simulink model "Quad_tilt_dynamic_fl"  (R2017b)
settings: Solver=FixedStepAuto  StartTime=0.0  StopTime=30  FixedStep=0.0001  RelTol=1e-3
values from neighbouring files (symbols this model uses):
  alpha1_0 = 0.0    (= 0)    [parameters_quad_tilt_dynamic.m]
  alpha2_0 = pi    (= 3.14159265359)    [parameters_quad_tilt_dynamic.m]
  alpha3_0 = 0.0    (= 0)    [parameters_quad_tilt_dynamic.m]
  alpha4_0 = pi    (= 3.14159265359)    [parameters_quad_tilt_dynamic.m]
  d2wd = zeros(3,1)    [parameters_quad_tilt_dynamic.m]
  dx0 = 0.0    (= 0)    [parameters_quad_tilt_dynamic.m]
  dy0 = 0.0    (= 0)    [parameters_quad_tilt_dynamic.m]
  dz0 = 1.0    (= 1)    [parameters_quad_tilt_dynamic.m]
  gravity = [0.0;0.0;-g]    [parameters_quad_tilt_dynamic.m]
  Inertia_Matrix = [Ix, 0,  0 ... (first row only)    [parameters_quad_tilt_dynamic.m]
  Inv_Iner = inv(Inertia_Matrix)    [parameters_quad_tilt_dynamic.m]
  K2d = eye(3) * 7.5    [parameters_quad_tilt_dynamic.m]
  Kd = eye(3) * 25.75    [parameters_quad_tilt_dynamic.m]
  kf = 0.3    [parameters_quad_tilt_dynamic.m]
  km = 0.1    [parameters_quad_tilt_dynamic.m]
  Kp = eye(3) * 15    [parameters_quad_tilt_dynamic.m]
  Kw = eye(3) * 10    [parameters_quad_tilt_dynamic.m]
  l = 0.1    [parameters_quad_tilt_dynamic.m]
  m = 0.650    (= 0.65)    [parameters_quad_tilt_dynamic.m]
  Rb0 = eye(3)    [parameters_quad_tilt_dynamic.m]
  Rd = [  1.0000000,  0.0000000,  0.0000000 ... (first row only)    [parameters_quad_tilt_dynamic.m]
  Wb0 = [0.0, 0.0, 0.0]    [parameters_quad_tilt_dynamic.m]
  x0 = 1.0    (= 1)    [parameters_quad_tilt_dynamic.m]
  y0 = 0.0    (= 0)    [parameters_quad_tilt_dynamic.m]
  z0 = 0.0    (= 0)    [parameters_quad_tilt_dynamic.m]
libraries: simulink x4
settings Model: Creator=Marco  LastModifiedBy=Marco
settings CodeAppCC: StateflowObjectComments=on

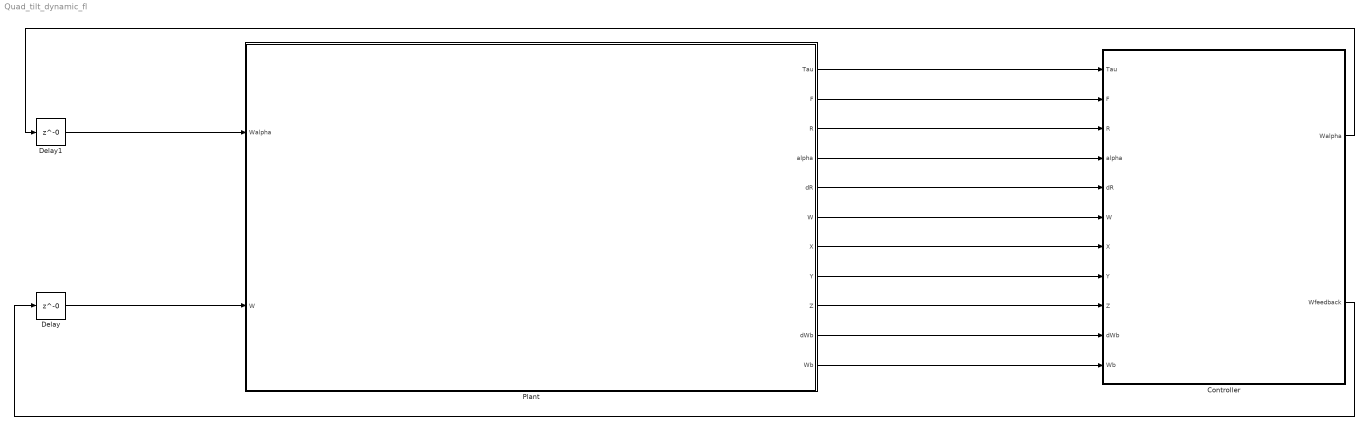
== system Quad_tilt_dynamic_fl ==
  Controller : Subsystem
  Delay : Delay  DelayLength=0  InitialCondition=zeros(4,1)
  Delay1 : Delay  DelayLength=0  InitialCondition=zeros(4,1)
  Plant : Subsystem
  wires:
  Delay/1 -> Plant/2(W)
  Delay1/1 -> Plant/1("Walpha ")
  Plant/1(Tau) -> Controller/1(Tau)
  Plant/2(F) -> Controller/2(F)
  Plant/3(R) -> Controller/3(R)
  Plant/4(alpha) -> Controller/4(alpha)
  Plant/6("W ") -> Controller/6(W)
  Plant/5(dR) -> Controller/5(dR)
  Plant/7(X) -> Controller/7(X)
  Plant/8(Y) -> Controller/8(Y)
  Plant/9(Z) -> Controller/9(Z)
  Controller/1(Walpha) -> Delay1/1
  Controller/2(Wfeedback) -> Delay/1
  Plant/10(dWb) -> Controller/10(dWb)
  Plant/11(Wb) -> Controller/11(Wb)

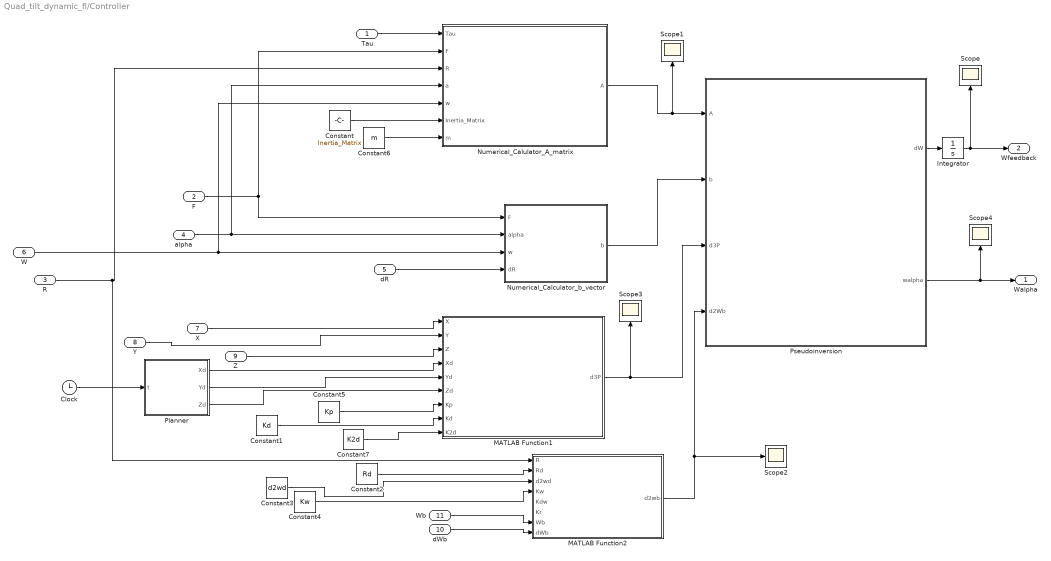
== system Quad_tilt_dynamic_fl/Controller ==
  Tau : Inport
  F : Inport  Port=2
  R : Inport  Port=3
  alpha : Inport  Port=4
  dR : Inport  Port=5
  W : Inport  Port=6
  X : Inport  Port=7
  Y : Inport  Port=8
  Z : Inport  Port=9
  dWb : Inport  Port=10
  Wb : Inport  Port=11
  Clock : Clock
  Constant : Constant  Value=Inertia_Matrix
  Constant1 : Constant  Value=Kd
  Constant2 : Constant  Value=Rd
  Constant3 : Constant  Value=d2wd
  Constant4 : Constant  Value=Kw
  Constant5 : Constant  Value=Kp
  Constant6 : Constant  Value=m
  Constant7 : Constant  Value=K2d
  Integrator : Integrator  InitialCondition=zeros(4,1)
  MATLAB Function1 : MATLAB Function  TreatAsAtomicUnit=on
  MATLAB Function2 : MATLAB Function  TreatAsAtomicUnit=on
  Numerical_Calculator_b_vector : MATLAB Function  TreatAsAtomicUnit=on
  Numerical_Calulator_A_matrix : MATLAB Function  TreatAsAtomicUnit=on
  Planner : MATLAB Function  TreatAsAtomicUnit=on
  Pseudoinversion : MATLAB Function  TreatAsAtomicUnit=on
  Scope{,1..4} (5 alike) : Scope
  Walpha : Outport
  Wfeedback : Outport  Port=2
  wires:
  Tau/1 -> Numerical_Calulator_A_matrix/1(Tau)
  alpha/1 -> Numerical_Calculator_b_vector/2(alpha), Numerical_Calulator_A_matrix/4(a)
  W/1 -> Numerical_Calculator_b_vector/3(w), Numerical_Calulator_A_matrix/5(w)
  R/1 -> MATLAB Function2/1(R), Numerical_Calulator_A_matrix/3(R)
  dR/1 -> Numerical_Calculator_b_vector/4(dR)
  F/1 -> Numerical_Calculator_b_vector/1(F), Numerical_Calulator_A_matrix/2(F)
  Constant/1 -> Numerical_Calulator_A_matrix/6(Inertia_Matrix)
  X/1 -> MATLAB Function1/1(X)
  Y/1 -> MATLAB Function1/2(Y)
  Z/1 -> MATLAB Function1/3(Z)
  Constant5/1 -> MATLAB Function1/7(Kp)
  Constant1/1 -> MATLAB Function1/8(Kd)
  Clock/1 -> Planner/1(t)
  Planner/1(Xd) -> MATLAB Function1/4(Xd)
  Planner/2(Yd) -> MATLAB Function1/5(Yd)
  Planner/3(Zd) -> MATLAB Function1/6(Zd)
  Constant3/1 -> MATLAB Function2/3(d2wd)
  Constant2/1 -> MATLAB Function2/2(Rd)
  Constant4/1 -> MATLAB Function2/4(Kw)
  Numerical_Calculator_b_vector/1(b) -> Pseudoinversion/2(b)
  Numerical_Calulator_A_matrix/1(A) -> Pseudoinversion/1(A), Scope1/1
  MATLAB Function1/1(d3P) -> Scope3/1, Pseudoinversion/3(d3P)
  Pseudoinversion/1(dW) -> Integrator/1
  Pseudoinversion/2(walpha) -> Scope4/1, Walpha/1
  Integrator/1 -> Scope/1, Wfeedback/1
  MATLAB Function2/1(d2wb) -> Scope2/1, Pseudoinversion/4(d2Wb)
  Constant6/1 -> Numerical_Calulator_A_matrix/7(m)
  Constant7/1 -> MATLAB Function1/9(K2d)
  Wb/1 -> MATLAB Function2/7(Wb)
  dWb/1 -> MATLAB Function2/8(dWb)

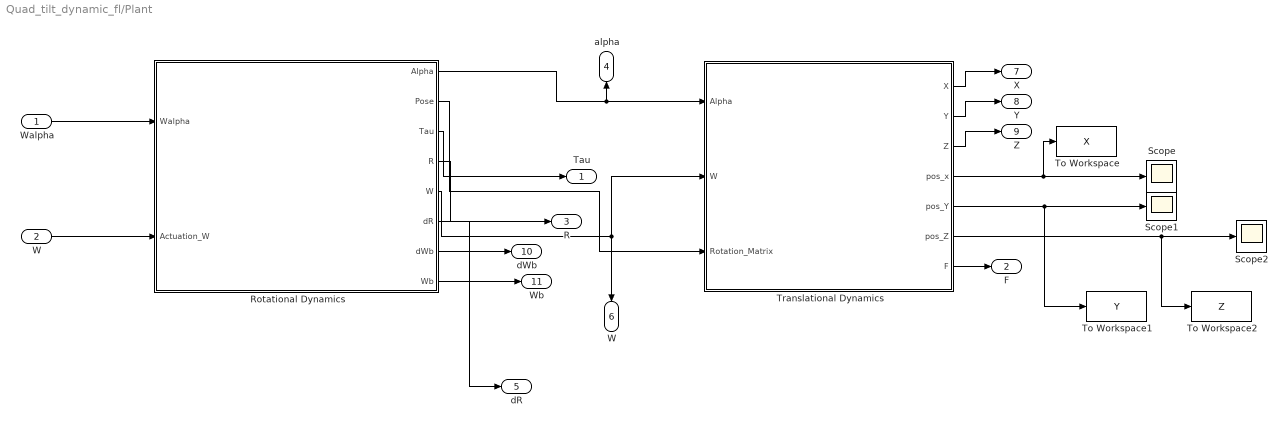
== system Quad_tilt_dynamic_fl/Plant ==
  "Walpha " : Inport
  W : Inport  Port=2
  Rotational Dynamics : Subsystem
  Scope : Scope
  Scope1 : Scope
  Scope2 : Scope
  To Workspace : ToWorkspace  VariableName=X  SampleTime=-1
  To Workspace1 : ToWorkspace  VariableName=Y  SampleTime=-1
  To Workspace2 : ToWorkspace  VariableName=Z  SampleTime=-1
  Translational Dynamics : Subsystem
  Tau : Outport
  F : Outport  Port=2
  R : Outport  Port=3
  alpha : Outport  Port=4
  dR : Outport  Port=5
  "W " : Outport  Port=6
  X : Outport  Port=7
  Y : Outport  Port=8
  Z : Outport  Port=9
  dWb : Outport  Port=10
  Wb : Outport  Port=11
  wires:
  Rotational Dynamics/3(Tau) -> Tau/1
  Rotational Dynamics/2(Pose) -> Translational Dynamics/3(Rotation_Matrix)
  Rotational Dynamics/1(Alpha) -> alpha/1, Translational Dynamics/1(Alpha)
  Translational Dynamics/7(F) -> F/1
  Translational Dynamics/1(X) -> X/1
  Translational Dynamics/2(Y) -> Y/1
  Translational Dynamics/3(Z) -> Z/1
  Rotational Dynamics/4(R) -> R/1
  "Walpha "/1 -> Rotational Dynamics/1(Walpha)
  W/1 -> Rotational Dynamics/2(Actuation_W)
  Rotational Dynamics/5(W) -> Translational Dynamics/2(W), "W "/1
  Translational Dynamics/4(pos_x) -> To Workspace/1, Scope/1
  Translational Dynamics/5(pos_Y) -> To Workspace1/1, Scope1/1
  Translational Dynamics/6(pos_Z) -> To Workspace2/1, Scope2/1
  Rotational Dynamics/6(dR) -> dR/1
  Rotational Dynamics/7(dWb) -> dWb/1
  Rotational Dynamics/8(Wb) -> Wb/1

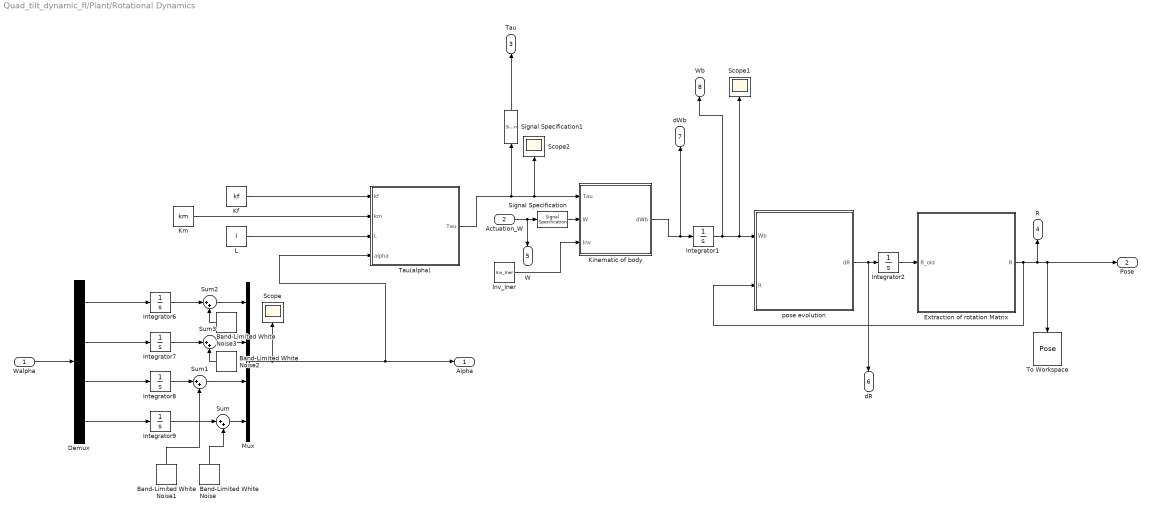
== system Quad_tilt_dynamic_fl/Plant/Rotational Dynamics ==
  Walpha : Inport
  Actuation_W : Inport  Port=2
  Band-Limited White Noise : simulink/Sources/Band-Limited White Noise  Cov=[0]  Ts=0.1  seed=[23345431]
  Band-Limited White Noise1 : simulink/Sources/Band-Limited White Noise  Cov=[0]  Ts=0.1  seed=[233423781]
  Band-Limited White Noise2 : simulink/Sources/Band-Limited White Noise  Cov=[0]  Ts=0.1  seed=[232441]
  Band-Limited White Noise3 : simulink/Sources/Band-Limited White Noise  Cov=[0]  Ts=0.1  seed=[23341]
  Demux : Demux
  Extraction of rotation Matrix : MATLAB Function  TreatAsAtomicUnit=on
  Integrator1 : Integrator  InitialCondition=Wb0
  Integrator2 : Integrator  InitialCondition=Rb0
  Integrator6 : Integrator  InitialCondition=alpha1_0
  Integrator7 : Integrator  InitialCondition=alpha2_0
  Integrator8 : Integrator  InitialCondition=alpha3_0
  Integrator9 : Integrator  InitialCondition=alpha4_0
  Inv_Iner : Constant  Value=Inv_Iner
  Kf : Constant  Value=kf
  Kinematic of body : MATLAB Function  TreatAsAtomicUnit=on
  Km : Constant  Value=km
  L : Constant  Value=l
  Mux : Mux
  Scope : Scope
  Scope1 : Scope
  Scope2 : Scope
  Signal Specification : SignalSpecification  Dimensions=[4,1]
  Signal Specification1 : SignalSpecification  Dimensions=[3,4]
  Sum{,1..3} (4 alike) : Sum  Inputs=|++
  Tau(alpha) : MATLAB Function  TreatAsAtomicUnit=on
  To Workspace : ToWorkspace  VariableName=Pose  SampleTime=-1
      settings: Save2DSignal=2-D array (concatenate along first dimension)
  pose evolution : MATLAB Function  TreatAsAtomicUnit=on
  Alpha : Outport
  Pose : Outport  Port=2
  Tau : Outport  Port=3
  R : Outport  Port=4
  W : Outport  Port=5
  dR : Outport  Port=6
  dWb : Outport  Port=7
  Wb : Outport  Port=8
  wires:
  Integrator9/1 -> Sum/1
  Kf/1 -> Tau(alpha)/1(kf)
  Demux/1 -> Integrator6/1
  Demux/2 -> Integrator7/1
  Tau(alpha)/1(Tau) -> Scope2/1, Kinematic of body/1(Tau), Signal Specification1/1
  Demux/3 -> Integrator8/1
  Demux/4 -> Integrator9/1
  L/1 -> Tau(alpha)/3(L)
  Km/1 -> Tau(alpha)/2(km)
  Integrator1/1 -> Scope1/1, pose evolution/1(Wb), Wb/1
  pose evolution/1(dR) -> dR/1, Integrator2/1
  Integrator2/1 -> Extraction of rotation Matrix/1(R_old)
  Extraction of rotation Matrix/1(R) -> R/1, Pose/1, To Workspace/1, pose evolution/2(R)
  Inv_Iner/1 -> Kinematic of body/3(Inv)
  Walpha/1 -> Demux/1
  Kinematic of body/1(dWb) -> dWb/1, Integrator1/1
  Mux/1 -> Scope/1, Tau(alpha)/4(alpha), Alpha/1
  Actuation_W/1 -> W/1, Signal Specification/1
  Signal Specification/1 -> Kinematic of body/2(W)
  Signal Specification1/1 -> Tau/1
  Band-Limited White Noise/1 -> Sum/2
  Sum/1 -> Mux/4
  Integrator8/1 -> Sum1/1
  Sum1/1 -> Mux/3
  Band-Limited White Noise1/1 -> Sum1/2
  Integrator6/1 -> Sum2/1
  Sum2/1 -> Mux/1
  Band-Limited White Noise3/1 -> Sum2/2
  Integrator7/1 -> Sum3/1
  Sum3/1 -> Mux/2
  Band-Limited White Noise2/1 -> Sum3/2

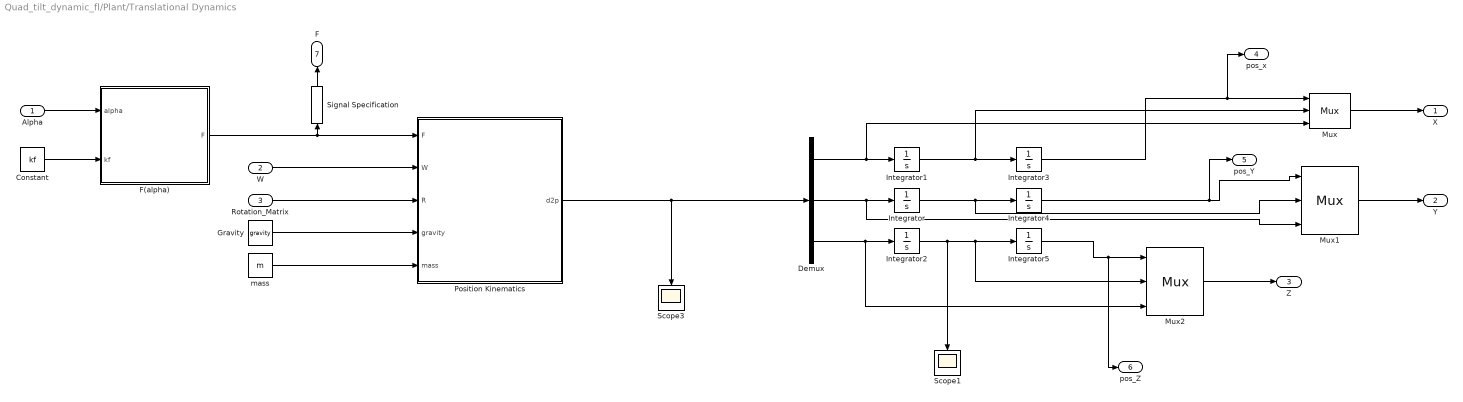
== system Quad_tilt_dynamic_fl/Plant/Translational Dynamics ==
  Alpha : Inport
  W : Inport  Port=2
  Rotation_Matrix : Inport  Port=3
  Constant : Constant  Value=kf
  Demux : Demux  Outputs=3
  F(alpha) : MATLAB Function  TreatAsAtomicUnit=on
  Gravity : Constant  Value=gravity
  Integrator : Integrator  InitialCondition=dy0
  Integrator1 : Integrator  InitialCondition=dx0
  Integrator2 : Integrator  InitialCondition=dz0
  Integrator3 : Integrator  InitialCondition=x0
  Integrator4 : Integrator  InitialCondition=y0
  Integrator5 : Integrator  InitialCondition=z0
  Mux : Mux  Inputs=3
  Mux1 : Mux  Inputs=3
  Mux2 : Mux  Inputs=3
  Position Kinematics : MATLAB Function  TreatAsAtomicUnit=on
  Scope1 : Scope
  Scope3 : Scope
  Signal Specification : SignalSpecification  Dimensions=[3,4]
  mass : Constant  Value=m
  X : Outport
  Y : Outport  Port=2
  Z : Outport  Port=3
  pos_x : Outport  Port=4
  pos_Y : Outport  Port=5
  pos_Z : Outport  Port=6
  F : Outport  Port=7
  wires:
  Demux/2 -> Mux1/3, Integrator/1
  Integrator4/1 -> pos_Y/1, Mux1/1
  Demux/3 -> Mux2/3, Integrator2/1
  Alpha/1 -> F(alpha)/1(alpha)
  Integrator/1 -> Mux1/2, Integrator4/1
  Integrator2/1 -> Scope1/1, Mux2/2, Integrator5/1
  Integrator3/1 -> pos_x/1, Mux/1
  Demux/1 -> Mux/3, Integrator1/1
  Constant/1 -> F(alpha)/2(kf)
  F(alpha)/1(F) -> Signal Specification/1, Position Kinematics/1(F)
  W/1 -> Position Kinematics/2(W)
  Rotation_Matrix/1 -> Position Kinematics/3(R)
  Gravity/1 -> Position Kinematics/4(gravity)
  mass/1 -> Position Kinematics/5(mass)
  Position Kinematics/1(d2p) -> Demux/1, Scope3/1
  Mux/1 -> X/1
  Mux1/1 -> Y/1
  Integrator5/1 -> pos_Z/1, Mux2/1
  Mux2/1 -> Z/1
  Integrator1/1 -> Mux/2, Integrator3/1
  Signal Specification/1 -> F/1

== matlab function Quad_tilt_dynamic_fl/Plant/Rotational Dynamics/Tau(alpha) ==
  data: kf input; km input; L input; alpha input; Tau output
function Tau = Tau_calc(kf,km,L,alpha)
    Tau = ones(3,4);
    s1 = sin(alpha(1));
    c1 = cos(alpha(1));
    s2 = sin(alpha(2));
    c2 = cos(alpha(2));
    s3 = sin(alpha(3));
    c3 = cos(alpha(3));
    s4 = sin(alpha(4));
    c4 = cos(alpha(4));
    Tau = [0,              -L*kf*c2 - km*s2,  0              , L*kf*c4+ km*s4;
          -L*kf*c1 + km*s1, 0              ,  L*kf*c3-km*s3  ,              0;
          -L*kf*s1 - km*c1, L*kf*s2-km*c2  , -L*kf*s3 - km*c3, L*kf*s4- km*c4];

== matlab function Quad_tilt_dynamic_fl/Plant/Translational Dynamics/F(alpha) ==
  data: alpha input; F output; kf input
function F = F(alpha,kf)
    F = ones(3,4);
    s1 = sin(alpha(1));
    c1 = cos(alpha(1));
    s2 = sin(alpha(2));
    c2 = cos(alpha(2));
    s3 = sin(alpha(3));
    c3 = cos(alpha(3));
    s4 = sin(alpha(4));
    c4 = cos(alpha(4));
    F(1,:) = [0, -s2, 0, s4];
    F(2,:) = [-s1, 0, s3, 0];
    F(3,:) = [c1, -c2, c3, -c4];
    F = F * kf;

== matlab function Quad_tilt_dynamic_fl/Plant/Rotational Dynamics/pose evolution ==
  data: Wb input; dR output; R input
function dR = dR(Wb,R)
S = [0,  -Wb(2),Wb(3);
     Wb(2),0,  -Wb(1);
     -Wb(3),Wb(1),0];
 dR = S * R;

== matlab function Quad_tilt_dynamic_fl/Plant/Rotational Dynamics/Extraction of rotation Matrix ==
  data: R output; R_old input
function R = extractionR(R_old)
    [U,Sigma,V] = svd(R_old);
    R = U*V';

== matlab function Quad_tilt_dynamic_fl/Plant/Rotational Dynamics/Kinematic of body ==
  data: Tau input; dWb output; W input; Inv input
function dWb = fcn(Tau,W,Inv)
    dWb = zeros(3,1);
    dWb = Inv * Tau * W;

== matlab function Quad_tilt_dynamic_fl/Plant/Translational Dynamics/Position Kinematics ==
  data: F input; W input; d2p output; R input; gravity input; mass input
function d2p = acceleration(F,W,R,gravity,mass)

    d2p =  (R*F*W)/mass + gravity;

== matlab function Quad_tilt_dynamic_fl/Controller/Numerical_Calulator_A_matrix ==
  data: Tau input; F input; A output; R input; a input; w input; Inertia_Matrix input; m input
function A = A_calculator(Tau,F,R,a,w,Inertia_Matrix,m)

%a corresponds to alpha
Jr = zeros(6,6);
Jr = [1/m * R,zeros(3,3);
      zeros(3,3),inv(Inertia_Matrix)];

J_bar = zeros(6,4);
J_bar = [F;Tau];

A = zeros(6,8);

dJ1 = zeros(6,4);
dJ2 = zeros(6,4);
dJ3 = zeros(6,4);
dJ4 = zeros(6,4);

dJ1 = [0, 0, 0, 0;
       -(3*cos(a(1)))/10, 0, 0, 0;
       -(3*sin(a(1)))/10, 0, 0, 0;
       0, 0, 0, 0;
       cos(a(1))/10 + (3*sin(a(1)))/100, 0, 0, 0;
       sin(a(1))/10 - (3*cos(a(1)))/100, 0, 0, 0];

dJ2 = [0, -(3*cos(a(2)))/10, 0, 0;
       0, 0, 0, 0;
       0, (3*sin(a(2)))/10, 0, 0;
       0, (3*sin(a(2)))/100 - cos(a(2))/10, 0, 0;
       0, 0, 0, 0;
       0, (3*cos(a(2)))/100 + sin(a(2))/10, 0, 0];
dJ3 = [0, 0, 0, 0;
       0, 0, (3*cos(a(3)))/10, 0;
       0, 0,  -(3*sin(a(3)))/10, 0;
       0, 0, 0, 0;
       0, 0, - cos(a(3))/10 - (3*sin(a(3)))/100, 0;
       0, 0,   sin(a(3))/10 - (3*cos(a(3)))/100, 0];
   
dJ4 = [0, 0, 0, (3*cos(a(4)))/10;
       0, 0, 0,  0;
       0, 0, 0,  (3*sin(a(4)))/10;
       0, 0, 0, cos(a(4))/10 - (3*sin(a(4)))/100;
       0, 0, 0, 0;
       0, 0, 0, (3*cos(a(4)))/100 + sin(a(4))/10];
A = Jr * [J_bar,dJ1*w(1) + dJ2 * w(2) + dJ3 * w(3) + dJ4 * w(4)];

== matlab function Quad_tilt_dynamic_fl/Controller/Numerical_Calculator_b_vector ==
  data: F input; b output; alpha input; w input; dR input
function b = b_calculator(F,alpha,w,dR)
b = zeros(6,1);
temp = dR * F * w;
b = [temp;zeros(3,1)];

== matlab function Quad_tilt_dynamic_fl/Controller/Planner ==
  data: t input; Xd output; Yd output; Zd output
function [Xd,Yd,Zd] = position_planner(t)
%Until third derivative of coordinates
%Xd = [0;0;0;0];
%Yd = [0;0;0;0];
%Zd = [0.0;0;0;0];
Xd = [cos(t);-sin(t);-cos(t);+sin(t)];
Yd = [0;0;0;0];
Zd = [sin(t);cos(t);-sin(t);-cos(t)];

== matlab function Quad_tilt_dynamic_fl/Controller/MATLAB Function1 ==
  data: X input; d3P output; Y input; Z input; Xd input; Yd input; Zd input; Kp input; Kd input; K2d input
function d3P  = Position_Error(X,Y,Z,Xd,Yd,Zd,Kp,Kd,K2d)
d3P = zeros(3,1);
ep = [Xd(1,1) - X(1,1);Yd(1,1) - Y(1,1);Zd(1,1) - Z(1,1)];
dep = [Xd(2,1) - X(2,1);Yd(2,1) - Y(2,1);Zd(2,1) - Z(2,1)];
d2ep = [Xd(3,1) - X(3,1);Yd(3,1) - Y(3,1);Zd(3,1) - Z(3,1)];
d3P = [Xd(4,1);Yd(4,1);Zd(4,1)] + Kp * ep + Kd * dep + K2d * d2ep;

== matlab function Quad_tilt_dynamic_fl/Controller/MATLAB Function2 ==
  data: R input; Rd input; d2wb output; d2wd input; Kw input; Kdw input; Kr input; Wb input; dWb input
function d2wb = error_rotation_matrix(R,Rd,d2wd,Kw,Kdw,Kr,Wb,dWb)
d2wb = zeros(3,1);
er = zeros(3,1);
A = zeros(3,3);
A = 0.5 * (R' * Rd - Rd' * R);
er = [A(3,2);A(2,1);-A(3,1)];
d2wb = d2wd + Kr * er - Kw * Wb - Kw * dWb;

== matlab function Quad_tilt_dynamic_fl/Controller/Pseudoinversion ==
  data: A input; dW output; b input; d3P input; d2Wb input; walpha output
function [dW,walpha] = pseudoinverse(A,b,d3P,d2Wb)
dW = zeros(4,1);
walpha = zeros(4,1);
C = zeros(8,1);
C = pinv(A) * ([d3P;d2Wb] - b);
dW = C(1:4,:);
walpha = C(5:8,:);
